simulink model "OneLeg_VR_TouchInput"  (Simulink 7.3)
settings: Solver=ode15s  StartTime=0.0  StopTime=inf  RelTol=1e-3
PreLoadFcn:
  | init_hopper
PostLoadFcn:
  | vrmfunc('FnOpen', [bdroot, '/Data Display and Analysis/VR Sink']);
undefined symbols (not defined in the file or in its folder): body, ctrl, ground, leg, sfuntraj, sigbuilder_block, Traj
libraries: mblibv1 x27, dspmtrx3 x8, simulink x4, vrlib x1
(part 1 of 2)
settings Model: Creator=grouleau  LastModifiedBy=grouleau
settings DataIOCC: SignalLoggingName=log
settings OptimizationCC: InitFltsAndDblsToZero=on
settings SimMechanicsCC: VisSampleTime=0.0667  AnimationDelay=0  LastVizWinPosition=[619 721 850 247]  CamPosition=[3.67411;0.656374;23.7815;]  CamTarget=[3.67411;0.656374;0;]  CamUpVector=[0;1;0;]  CamHeight=2.15758  VisBackgroundColor=[0.9;0.9;0.95;]  DefaultBodyColor=[1;0;0;]

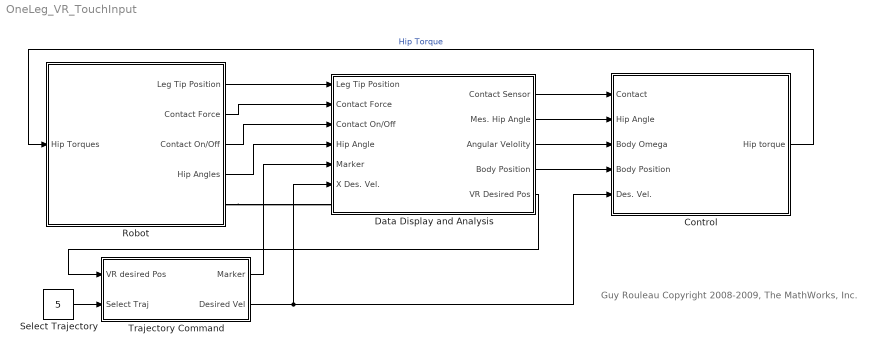
== system OneLeg_VR_TouchInput ==
  note: Guy Rouleau
      | Copyright 2008-2009, The MathWorks, Inc.
  Control : Subsystem
  Data Display and Analysis : Subsystem
  Robot : Subsystem
  Select Trajectory : Constant  Value=5  OutDataType=sfix(16)  OutScaling=2^0
  Trajectory Command : Subsystem
  wires:
  Robot/1(Leg Tip Position) -> Data Display and Analysis/1(Leg Tip Position)
  Control/1(Hip torque) -> Robot/1(Hip Torques)  "Hip Torque"
  Data Display and Analysis/3(Angular Velolity) -> Control/3(Body Omega)
  Robot/4(Hip Angles) -> Data Display and Analysis/4(Hip Angle)
  Trajectory Command/2(Desired Vel) -> Data Display and Analysis/6(X Des. Vel.), Control/5(Des. Vel.)
  Data Display and Analysis/4(Body Position) -> Control/4(Body Position)
  Data Display and Analysis/2(Mes. Hip Angle) -> Control/2(Hip Angle)
  Trajectory Command/1(Marker) -> Data Display and Analysis/5(Marker)
  Select Trajectory/1 -> Trajectory Command/2(Select Traj)
  Robot/3(Contact On/Off) -> Data Display and Analysis/3(Contact On/Off)
  Robot/2(Contact Force) -> Data Display and Analysis/2(Contact Force)
  Data Display and Analysis/5(VR Desired Pos) -> Trajectory Command/1(VR desired Pos)
  Data Display and Analysis/1(Contact Sensor) -> Control/1(Contact)
  connections:
  Robot/RConn1 -- Data Display and Analysis/LConn1

== system OneLeg_VR_TouchInput/Control ==
  Contact : Inport
  Hip Angle : Inport  Port=2
  Body Omega : Inport  Port=3
  Body Position : Inport  Port=4
  Des. Vel. : Inport  Port=5
  Body Angle Control : Subsystem
  Integrator : Integrator  LimitOutput=on  UpperSaturationLimit=1  LowerSaturationLimit=-1
  Logical Operator1 : Logic  Operator=NOT  AllPortsSameDT=off  OutDataTypeMode=boolean  OutDataTypeStr=boolean
  Motion analysis : Subsystem
  Saturation : Saturate  UpperLimit=ctrl.MaxHipTorque  LowerLimit=-ctrl.MaxHipTorque  OutDataType=sfix(16)  OutScaling=2^0
  Switch : Switch  Criteria=u2 ~= 0  OutDataType=sfix(16)  OutScaling=2^0
  Velocity Control : Subsystem
  Hip torque : Outport
  wires:
  Contact/1 -> Motion analysis/1(Contact), Switch/2, Logical Operator1/1, Body Angle Control/Enable
  Motion analysis/4(X stance) -> Velocity Control/4(X stance)
  Motion analysis/3(Body Vel) -> Velocity Control/3(Body Vel)
  Saturation/1 -> Hip torque/1
  Motion analysis/2(T up) -> Velocity Control/2(Air Duration)
  Hip Angle/1 -> Motion analysis/2(Hip Angle)
  Integrator/1 -> Motion analysis/3(Body Angle)
  Motion analysis/5(Leg Length) -> Velocity Control/5(Leg Length)
  Motion analysis/6(Hip Angle o) -> Velocity Control/6(Hip Angle)
  Motion analysis/1(Body Angle o) -> Body Angle Control/1(Theta), Velocity Control/1(Body Angle)
  Logical Operator1/1 -> Velocity Control/Enable
  Switch/1 -> Saturation/1
  Body Angle Control/1(Cmd) -> Switch/1
  Body Omega/1 -> Body Angle Control/2(Omega body), Integrator/1
  Velocity Control/1(Cmd) -> Switch/3
  Des. Vel./1 -> Motion analysis/4(Des. Vel.)
  Body Position/1 -> Motion analysis/5(Body Position)
  Motion analysis/7(Comp Des. Vel.) -> Velocity Control/7(Desired Velocity)
  Motion analysis/8(Comp Des. Pos.) -> Velocity Control/8(Desired Position)
  Motion analysis/9(Comp Body Pos.) -> Velocity Control/9(Body Pos)

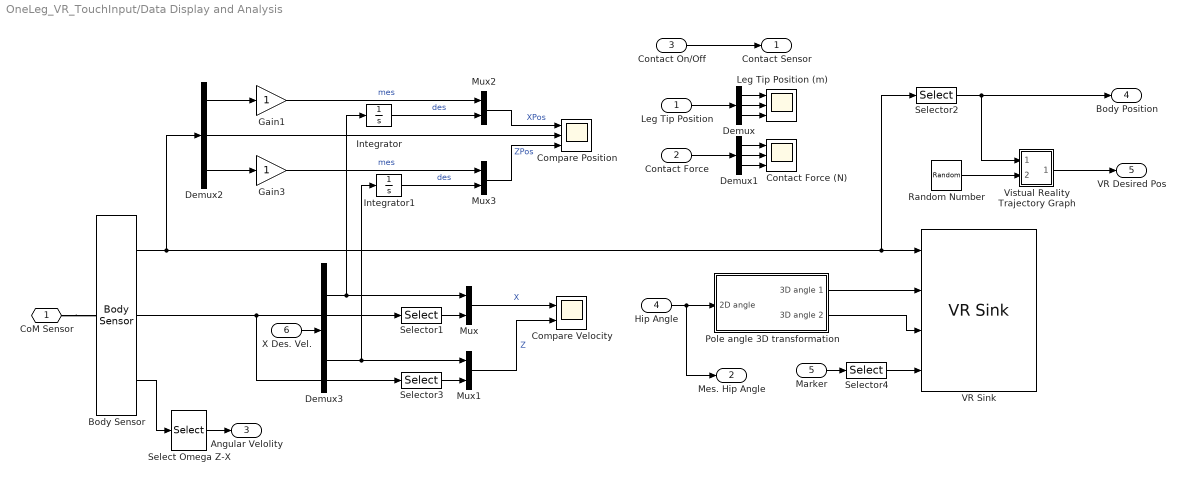
== system OneLeg_VR_TouchInput/Data Display and Analysis ==
  Leg Tip Position : Inport
  Contact Force : Inport  Port=2
  Contact On/Off : Inport  Port=3
  Hip Angle : Inport  Port=4
  Marker : Inport  Port=5
  X Des. Vel. : Inport  Port=6
  Body Sensor : mblibv1/Sensors &  Actuators/Body Sensor  DialogController=MECH.DynMechDlgSource  SystemSampleTime=-1  UpdateFromCAD=off  PhysicalDomain=Mechanical  PortType=blob  Muxed=off  Pose=off  Angle=on  AngleUnits=deg  ArcVelocity=on  ArcVelocityUnits=rad/s  ArcAcceleration=off  ArcAccelerationUnits=deg/s^2  CoordPosition=on  CoordPositionUnits=m  Velocity=on  VelocityUnits=m/s  Acceleration=off  AccelerationUnits=m/s^2  Quaternion=on  QuaternionDT=off  QuaternionDDT=off  QuaternionUnits=off  OutputVector=[1]  ActiveIO=on  Width=9  DialogClass=MechanicalSensorBlock  ReferenceFrame=Absolute (World)
  Compare Position : Scope  NumInputPorts=3
      settings: TimeRange=60  YMin=0~0.6~-1  YMax=4~1.15~1  SaveName=BodyData
  Compare Velocity : Scope  NumInputPorts=2
      settings: TimeRange=60  YMin=0.65~-1  YMax=1.2~1  SaveName=ScopeData10
  Contact Force (N) : Scope  NumInputPorts=3
      settings: TimeRange=2.5  YMin=-60000~0~-1  YMax=20000~20000~1
  Demux : Demux  Outputs=3
  Demux1 : Demux  Outputs=3
  Demux2 : Demux  Outputs=3
  Demux3 : Demux  Outputs=2
  Gain1 : Gain  ParameterDataType=sfix(16)  ParameterScaling=2^0  OutDataType=sfix(16)  OutScaling=2^0
  Gain3 : Gain  ParameterDataType=sfix(16)  ParameterScaling=2^0  OutDataType=sfix(16)  OutScaling=2^0
  Integrator : Integrator
  Integrator1 : Integrator
  Leg Tip Position (m) : Scope  NumInputPorts=3
      settings: YMin=-1~-0.05~-1  YMax=1~0.25~1  SaveName=FootData1
  Mux{,1..3} (4 alike) : Mux  Inputs=2
  Pole angle 3D transformation : Subsystem
  Random Number : RandomNumber  Mean=[0 0]  Variance=[5 5]  Seed=[0 5]  SampleTime=3
  Select Omega Z-X : Selector  InputPortWidth=3  IndexOptions=Index vector (dialog)  Indices=[3 1]  OutputSizes=1
  Selector1 : Selector  InputPortWidth=3  IndexOptions=Index vector (dialog)  Indices=[1 ]  OutputSizes=1
  Selector2 : Selector  InputPortWidth=3  IndexOptions=Index vector (dialog)  Indices=[1 3 ]  OutputSizes=1
  Selector3 : Selector  InputPortWidth=3  IndexOptions=Index vector (dialog)  Indices=[3 ]  OutputSizes=1
  Selector4 : Selector  InputPortWidth=3  IndexOptions=Index vector (dialog)  Indices=[1 3 2 ]  OutputSizes=1
  VR Sink : vrlib/VR Sink  InstantiateOnLoad=on  SampleTime=1/15  ViewEnable=on  RemoteChange=off  RemoteView=off  FieldsWritten=Pendulum.translation.3.1.double#Pole1.rotation.4.1.double#Pole2.rotation.4.1.double#Marker.translation.3.1.double  WorldFileName=robotVR.wrl  WorldDescription=Hopping Robot  AutoView=off  VideoDimensions=[]  FigureProperties="{'Position', 'Name', 'Viewpoint', 'CameraBound', 'CameraDirection', 'CameraPosition', 'CameraUpVector', 'ZoomFactor', 'Antialiasing', 'Headlight', 'Lighting', 'NavPanel', 'StatusBar', 'ToolBar', 'Textures', 'Transparency', 'Wireframe', 'NavZones', 'NavMode', 'NavSpeed', 'Record2DCompressMethod', 'Record2DCompressQuality', 'Record2D', 'Record2DFileName', 'Record2DFPS'; [5.0000000000000000e+000  9.2000000000000000e+001  5.7600000000000000e+002  3.8000000000000000e+002], 'Hopping Robot', 'Close view', 'on', [0.0000000000000000e+000  0.0000000000000000e+000 -1.0000000000000000e+000], [0.0000000000000000e+000  0.0000000000000000e+000  0.0000000000000000e+000], [0.0000000000000000e+000  1.0000000000000000e+000  0.0000000000000000e+000], [1.0000000000000000e+000], 'off', 'on', 'on', 'halfbar', 'on', 'on', 'on', 'on', 'off', 'off', 'examine', 'normal', 'auto', [7.5000000000000000e+001], 'off', '%f_anim_%n.avi', [1.5000000000000000e+001]}"
  Vistual Reality Trajectory Graph : Subsystem  LoadFcn=sfuntraj([],[],[],'LoadBlock')  StartFcn=sfuntraj([],[],[],'Start')  StopFcn=sfuntraj([],[],[],'Stop')  mask(Trajectory scope.){xmin=-10, xmax=10, ymin=-10, ymax=10, Ts=0.2, mode=VR sensor}
      mask prompts: xmin "x-min:"; xmax "x-max:"; ymin "y-min:"; ymax "y-max:"; Ts "Sample time:"; mode "Setpoint mode"
      mask help: Trajectory scope using MATLAB graph window. Enter plotting ranges.
      settings: CopyFcn=sfuntraj([],[],[],'CopyBlock')  DeleteFcn=sfuntraj([],[],[],'DeleteBlock')  NameChangeFcn=sfuntraj([],[],[],'NameChange')
      mask Help: This block can be used to explore limit cycles. Look at the m-file sfuntraj.m to see how it works.
      mask StyleString: edit,edit,edit,edit,edit,popup(Mouse|Input signal|VR sensor)
      mask Display: plot([.05 .95 .95 .05 .05],[.45 .45 .95 .95 .45], 0.5+cos(0:0.1:2*pi)*0.3,0.7+sin(0:0.1:2*pi)*0.2)
  CoM Sensor : PMIOPort  Port=1  Side=Left
  Contact Sensor : Outport
  Mes. Hip Angle : Outport  Port=2
  Angular Velolity : Outport  Port=3
  Body Position : Outport  Port=4
  VR Desired Pos : Outport  Port=5
  wires:
  Mux/1 -> Compare Velocity/1  "X"
  Selector1/1 -> Mux/2
  Body Sensor/2 -> Selector1/1, Selector3/1
  Mux1/1 -> Compare Velocity/2  "Z"
  Selector3/1 -> Mux1/2
  Body Sensor/1 -> Demux2/1, VR Sink/1, Selector2/1
  Demux3/1 -> Mux/1, Integrator/1
  Demux3/2 -> Mux1/1, Integrator1/1
  Body Sensor/3 -> Select Omega Z-X/1
  Hip Angle/1 -> Pole angle 3D transformation/1(2D angle), Mes. Hip Angle/1
  Pole angle 3D transformation/1(3D angle 1) -> VR Sink/2
  Pole angle 3D transformation/2(3D angle 2) -> VR Sink/3
  Marker/1 -> Selector4/1
  Integrator/1 -> Mux2/2  "des"
  Demux2/1 -> Gain1/1
  Integrator1/1 -> Mux3/2  "des"
  Demux2/3 -> Gain3/1
  Demux2/2 -> Compare Position/2
  Mux2/1 -> Compare Position/1  "XPos"
  Mux3/1 -> Compare Position/3  "ZPos"
  Gain1/1 -> Mux2/1  "mes"
  Gain3/1 -> Mux3/1  "mes"
  Selector2/1 -> Body Position/1, Vistual Reality Trajectory Graph/1(data)
  Select Omega Z-X/1 -> Angular Velolity/1
  Selector4/1 -> VR Sink/4
  Demux/1 -> Leg Tip Position (m)/1
  Demux/2 -> Leg Tip Position (m)/2
  Demux/3 -> Leg Tip Position (m)/3
  Leg Tip Position/1 -> Demux/1
  Contact Force/1 -> Demux1/1
  Demux1/1 -> Contact Force (N)/1
  Demux1/2 -> Contact Force (N)/2
  Demux1/3 -> Contact Force (N)/3
  X Des. Vel./1 -> Demux3/1
  Contact On/Off/1 -> Contact Sensor/1
  Random Number/1 -> Vistual Reality Trajectory Graph/2(setpoint)
  Vistual Reality Trajectory Graph/1(mouse) -> VR Desired Pos/1
  connections:
  CoM Sensor/RConn1 -- Body Sensor/LConn1

== system OneLeg_VR_TouchInput/Robot ==
  Hip Torques : Inport
  Body : Subsystem
  Hip : Subsystem
  Leg : mblibv1/Bodies/Body  DialogController=MECH.DynMechDlgSource  PhysicalDomain=mechanical  SubClassName=Unknown  LeftPortType=workingframe  RightPortType=workingframe  LConnTagsString=CS1  RConnTagsString=CS2  UpdateFromCAD=off  DialogClass=MechanicalBodyBlock  Mass=leg.mass  MassUnits=kg  InertiaUnits=kg*m^2  Inertia=leg.inertia  Shape=Cylinder  ShapeDims=[1 1]  ShapeUnits=m  ShapeUse=false  Density=1  DensityUnits=kg/m^3  DensityUse=false  GraphicsMode=1  BodyColorSelMode=MACHINE_DEFAULT  BodyColor=[0.5 0.5 0.5]  AttachedToCS=1  CG="Left$CG$[0 -leg.length/3  0]$CS1$CS1$m$[0 0 0]$Euler X-Y-Z$rad$Adjoining$false$none"  WorkingFrames=Left$CS1$[0 0 0]$Adjoining$Adjoining$m$[0 0 0]$Euler X-Y-Z$deg$CG$true$none#Right$CS2$[0 -leg.length 0]$CS1$CS1$m$[0 0 0]$Euler X-Y-Z$deg$CS1$true$none  CGPos="[0 -leg.length/3  0]"  CGRot=[0 0 0]  CS0Pos=[]  CS0Rot=[]  CS1Pos=[0 0 0]  CS1Rot=[0 0 0]  CS2Pos=[0 -leg.length 0]  CS2Rot=[0 0 0]  CS3Pos=[]  CS3Rot=[]  CS4Pos=[]  CS4Rot=[]  CS5Pos=[]  CS5Rot=[]  CS6Pos=[]  CS6Rot=[]  CS7Pos=[]  CS7Rot=[]  CS8Pos=[]  CS8Rot=[]  CS9Pos=[]  CS9Rot=[]  CS10Pos=[]  CS10Rot=[]  CS11Pos=[]  CS11Rot=[]  CS12Pos=[]  CS12Rot=[]  CS13Pos=[]  CS13Rot=[]  CS14Pos=[]  CS14Rot=[]  CS15Pos=[]  CS15Rot=[]  CS16Pos=[]  CS16Rot=[]  CS17Pos=[]  CS17Rot=[]  CS18Pos=[]  CS18Rot=[]  CS19Pos=[]  CS19Rot=[]  CS20Pos=[]  CS20Rot=[]
  Leg Tip and Contact Dynamics : Subsystem
  Simplified Hydraulic Actuator : Subsystem
  Spring : Subsystem
  ComSensor : PMIOPort  Port=1  Side=Right
  Leg Tip Position : Outport
  Contact Force : Outport  Port=2
  Contact On/Off : Outport  Port=3
  Hip Angles : Outport  Port=4
  wires:
  Spring/1(Length) -> Simplified Hydraulic Actuator/1(Spring Length)
  Hip Torques/1 -> Hip/1(Torques)
  Hip/1(Hip Angles) -> Hip Angles/1
  Leg Tip and Contact Dynamics/1(Pos) -> Leg Tip Position/1
  Leg Tip and Contact Dynamics/2(Contact Force2) -> Contact Force/1  "Force (N)"
  Leg Tip and Contact Dynamics/3(Contact) -> Contact On/Off/1  "Contact"
  connections:
  Body/RConn1 -- Hip/LConn1
  Hip/RConn1 -- Leg/LConn1
  Leg/RConn1 -- Simplified Hydraulic Actuator/LConn1
  Spring/RConn1 -- Leg Tip and Contact Dynamics/LConn1
  Simplified Hydraulic Actuator/RConn1 -- Spring/LConn1
  ComSensor/RConn1 -- Body/RConn2

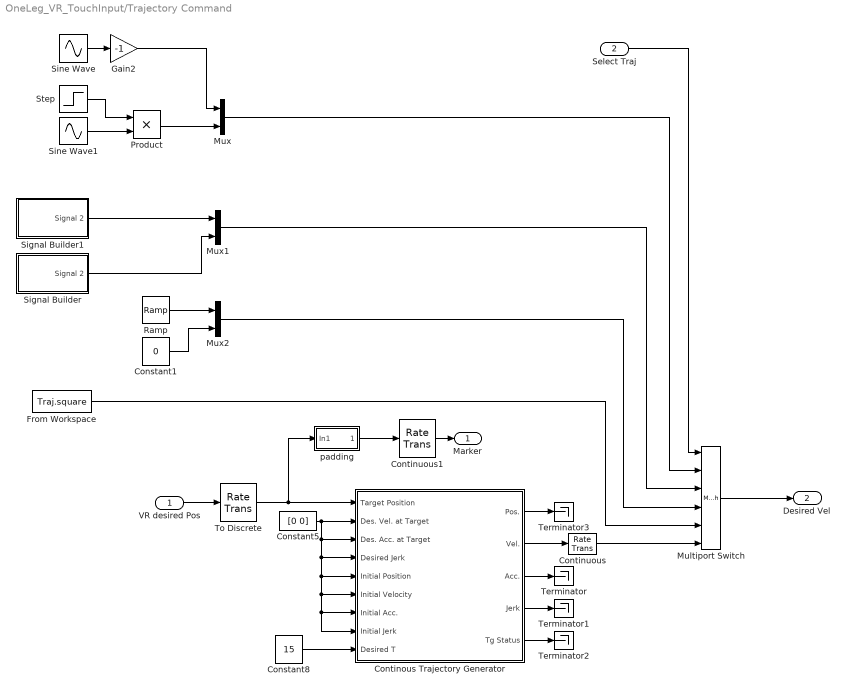
== system OneLeg_VR_TouchInput/Trajectory Command ==
  VR desired Pos : Inport  OutDataType=sfix(16)  OutScaling=2^0
  Select Traj : Inport  Port=2  OutDataType=sfix(16)  OutScaling=2^0
  Constant1 : Constant  Value=0  OutDataType=sfix(16)  OutScaling=2^0
  Constant5 : Constant  Value=[0 0]  OutDataType=sfix(16)  OutScaling=2^0  SampleTime=.01
  Constant8 : Constant  Value=15  OutDataType=sfix(16)  OutScaling=2^0  SampleTime=.01
  Continous Trajectory Generator : Subsystem  mask(Discrete Trajectory Generator: 5th Order Polynomial){UpdateLimit=0.0001, max_acc=50, maxv=.25, st=.01, Synchro=on}
      mask prompts: UpdateLimit "Treshold for Trajectory Update"; max_acc "Maximum acceleration"; maxv "Maximum velocity"; st "Sample time"; Synchro "Activate Synchronization"
      mask help:
      | Generates a 5th order polynomial trajectory between the current output and the desired position, velocity and acceleration. The motion will be executed in the requested trajectory time.
      | - The trajectory is updated when desired position changes
      | - This blocks accepts vectorized inputs.
      | - The input signals should have the same sampling time as the block.
      | - The motion will start one time step after the block is enabled and will be completed within the requested time if possible.
      mask Display: disp('7th Order\nPolynomial')
  Continuous : RateTransition  OutPortSampleTime=0
  Continuous1 : RateTransition  OutPortSampleTime=0
  From Workspace : FromWorkspace  VariableName=Traj.square  SampleTime=0  OutputAfterFinalValue=Holding final value
  Gain2 : Gain  Gain=-1  ParameterDataType=sfix(16)  ParameterScaling=2^0  OutDataType=sfix(16)  OutScaling=2^0
  Multiport Switch : MultiPortSwitch  Inputs=5  OutDataType=sfix(16)  OutScaling=2^0
  Mux : Mux  Inputs=2
  Mux1 : Mux  Inputs=2
  Mux2 : Mux  Inputs=2
  Product : Product  OutDataType=sfix(16)  OutScaling=2^0  RndMeth=Zero
  Ramp : simulink/Sources/Ramp  SystemSampleTime=-1  slope=.01  start=5  X0=0
  Signal Builder : Subsystem  Tag=STV Subsys  LoadFcn=sigbuilder_block('load');  StartFcn=sigbuilder_block('start');  StopFcn=sigbuilder_block('stop');  ClipboardFcn=sigbuilder_block('clipboard');  mask(Sigbuilder block){}
      mask help: Sigbuilder GUI
      mask init:
      | if ~strcmp(get_param(bdroot(gcbh),'SimulationStatus'),'stopped') tuvar = sigbuilder_block('maskInit'); end
      settings: CopyFcn=sigbuilder_block('copy');  DeleteFcn=sigbuilder_block('delete');  ModelCloseFcn=sigbuilder_block('modelClose');  PreSaveFcn=sigbuilder_block('preSave');  NameChangeFcn=sigbuilder_block('namechange');  OpenFcn=sigbuilder_block('open',[537.75 129 550.5 399.75 ]);  CloseFcn=sigbuilder_block('close');
      mask Display: plot(0,0,100,100,[10,10,40,40,10],[80,20,20,80,80],[40,10],[50,50], [40,27,10],[65,72,56],[40,25,25,10],[28,28,43,43]);
  Signal Builder1 : Subsystem  Tag=STV Subsys  LoadFcn=sigbuilder_block('load');  StartFcn=sigbuilder_block('start');  StopFcn=sigbuilder_block('stop');  ClipboardFcn=sigbuilder_block('clipboard');  mask(Sigbuilder block){}
      mask help: Sigbuilder GUI
      mask init:
      | if ~strcmp(get_param(bdroot(gcbh),'SimulationStatus'),'stopped') tuvar = sigbuilder_block('maskInit'); end
      settings: CopyFcn=sigbuilder_block('copy');  DeleteFcn=sigbuilder_block('delete');  ModelCloseFcn=sigbuilder_block('modelClose');  PreSaveFcn=sigbuilder_block('preSave');  NameChangeFcn=sigbuilder_block('namechange');  OpenFcn=sigbuilder_block('open',[537.75 129 550.5 399.75 ]);  CloseFcn=sigbuilder_block('close');
      mask Display: plot(0,0,100,100,[10,10,40,40,10],[80,20,20,80,80],[40,10],[50,50], [40,27,10],[65,72,56],[40,25,25,10],[28,28,43,43]);
  Sine Wave : Sin  Amplitude=Traj.circle.A  Bias=0  Frequency=Traj.circle.omega  Phase=0  Samples=10  SampleTime=0  Offset=0
  Sine Wave1 : Sin  Amplitude=Traj.circle.A  Bias=0  Frequency=Traj.circle.omega  Phase=pi/2  Samples=10  SampleTime=0  Offset=0
  Step : Step  Time=Traj.circle.starttime  SampleTime=0
  Terminator{,1..3} (4 alike) : Terminator
  To Discrete : RateTransition  OutPortSampleTime=.01
  padding : Subsystem
  Marker : Outport
  Desired Vel : Outport  Port=2
  wires:
  Sine Wave/1 -> Gain2/1
  Sine Wave1/1 -> Product/2
  Step/1 -> Product/1
  Gain2/1 -> Mux/1
  Signal Builder1/1(Signal 2) -> Mux1/1
  Signal Builder/1(Signal 2) -> Mux1/2
  Product/1 -> Mux/2
  Multiport Switch/1 -> Desired Vel/1
  Select Traj/1 -> Multiport Switch/1
  Mux/1 -> Multiport Switch/2
  Ramp/1 -> Mux2/1
  Constant1/1 -> Mux2/2
  Mux2/1 -> Multiport Switch/4
  Mux1/1 -> Multiport Switch/3
  From Workspace/1 -> Multiport Switch/5
  Constant5/1 -> Continous Trajectory Generator/2(Des. Vel. at Target), Continous Trajectory Generator/3(Des. Acc. at Target), Continous Trajectory Generator/4(Desired Jerk), Continous Trajectory Generator/5(Initial Position), Continous Trajectory Generator/6(Initial Velocity), Continous Trajectory Generator/7(Initial Acc.), Continous Trajectory Generator/8(Initial Jerk)
  Constant8/1 -> Continous Trajectory Generator/9(Desired T)
  Continous Trajectory Generator/2(Vel.) -> Continuous/1
  Continous Trajectory Generator/3(Acc.) -> Terminator/1
  Continous Trajectory Generator/4(Jerk) -> Terminator1/1
  Continous Trajectory Generator/5(Tg Status) -> Terminator2/1
  Continous Trajectory Generator/1(Pos.) -> Terminator3/1
  Continuous/1 -> Multiport Switch/6
  VR desired Pos/1 -> To Discrete/1
  padding/1(Out1) -> Continuous1/1
  Continuous1/1 -> Marker/1
  To Discrete/1 -> padding/1(In1), Continous Trajectory Generator/1(Target Position)

== system OneLeg_VR_TouchInput/Control/Body Angle Control ==
  Theta : Inport
  Omega body : Inport  Port=2
  Enable : EnablePort
  Omega Gain : Gain  Gain=ctrl.angle.Kv  ParameterDataType=sfix(16)  ParameterScaling=2^0  OutDataType=sfix(16)  OutScaling=2^0
  Position Gain : Gain  Gain=ctrl.angle.Kp  ParameterDataType=sfix(16)  ParameterScaling=2^0  OutDataType=sfix(16)  OutScaling=2^0
  Sum6 : Sum  Inputs=|++  OutDataType=sfix(16)  OutScaling=2^0
  Cmd : Outport
  wires:
  Sum6/1 -> Cmd/1
  Omega body/1 -> Omega Gain/1
  Theta/1 -> Position Gain/1
  Omega Gain/1 -> Sum6/2
  Position Gain/1 -> Sum6/1

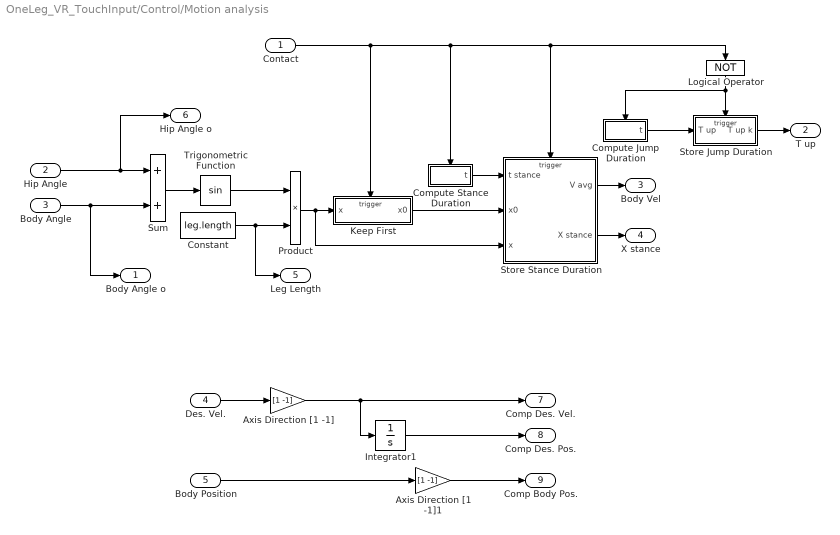
== system OneLeg_VR_TouchInput/Control/Motion analysis ==
  Contact : Inport
  Hip Angle : Inport  Port=2
  Body Angle : Inport  Port=3
  Des. Vel. : Inport  Port=4
  Body Position : Inport  Port=5
  Axis Direction [1 -1] : Gain  Gain=[1 -1]  ParameterDataType=sfix(16)  ParameterScaling=2^0  OutDataType=sfix(16)  OutScaling=2^0
  Axis Direction [1 -1]1 : Gain  Gain=[1 -1]  ParameterDataType=sfix(16)  ParameterScaling=2^0  OutDataType=sfix(16)  OutScaling=2^0
  Compute Jump Duration : Subsystem
  Compute Stance Duration : Subsystem
  Constant : Constant  Value=leg.length  OutDataType=sfix(16)  OutScaling=2^0
  Integrator1 : Integrator
  Keep First : Subsystem  TreatAsAtomicUnit=on
  Logical Operator : Logic  Operator=NOT  AllPortsSameDT=off  OutDataTypeMode=boolean  OutDataTypeStr=boolean
  Product : Product  OutDataType=sfix(16)  OutScaling=2^0  RndMeth=Zero
  Store Jump Duration : Subsystem  TreatAsAtomicUnit=on
  Store Stance Duration : Subsystem  TreatAsAtomicUnit=on
  Sum : Sum  OutDataType=sfix(16)  OutScaling=2^0
  Trigonometric Function : Trigonometry
  Body Angle o : Outport
  T up : Outport  Port=2
  Body Vel : Outport  Port=3
  X stance : Outport  Port=4
  Leg Length : Outport  Port=5
  Hip Angle o : Outport  Port=6
  Comp Des. Vel. : Outport  Port=7
  Comp Des. Pos. : Outport  Port=8
  Comp Body Pos. : Outport  Port=9
  wires:
  Hip Angle/1 -> Hip Angle o/1, Sum/1
  Body Angle/1 -> Body Angle o/1, Sum/2
  Sum/1 -> Trigonometric Function/1
  Trigonometric Function/1 -> Product/1
  Product/1 -> Keep First/1(x), Store Stance Duration/3(x)
  Keep First/1(x0) -> Store Stance Duration/2(x0)
  Compute Stance Duration/1(t) -> Store Stance Duration/1(t stance)
  Logical Operator/1 -> Compute Jump Duration/Enable, Store Jump Duration/Trigger
  Compute Jump Duration/1(t) -> Store Jump Duration/1(T up)
  Contact/1 -> Keep First/Trigger, Compute Stance Duration/Enable, Logical Operator/1, Store Stance Duration/Trigger
  Store Jump Duration/1(T up k) -> T up/1
  Store Stance Duration/1(V avg) -> Body Vel/1
  Store Stance Duration/2(X stance) -> X stance/1
  Constant/1 -> Product/2, Leg Length/1
  Des. Vel./1 -> Axis Direction [1 -1]/1
  Body Position/1 -> Axis Direction [1 -1]1/1
  Axis Direction [1 -1]/1 -> Integrator1/1, Comp Des. Vel./1
  Integrator1/1 -> Comp Des. Pos./1
  Axis Direction [1 -1]1/1 -> Comp Body Pos./1

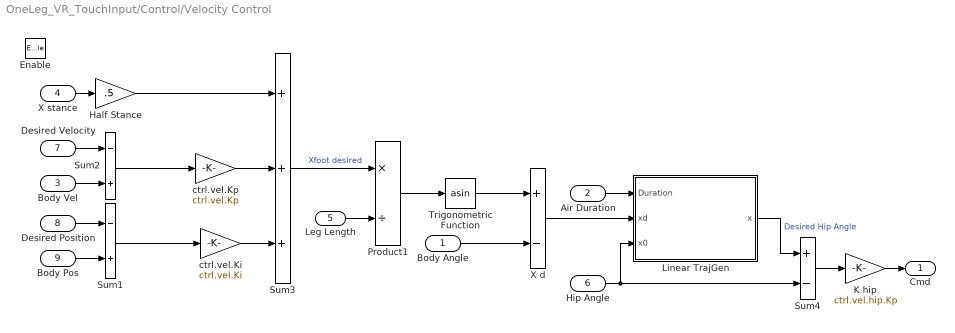
== system OneLeg_VR_TouchInput/Control/Velocity Control ==
  Body Angle : Inport
  Air Duration : Inport  Port=2
  Body Vel : Inport  Port=3
  X stance : Inport  Port=4
  Leg Length : Inport  Port=5
  Hip Angle : Inport  Port=6
  Desired Velocity : Inport  Port=7
  Desired Position : Inport  Port=8
  Body Pos : Inport  Port=9
  Enable : EnablePort  StatesWhenEnabling=reset
  Half Stance : Gain  Gain=.5  ParameterDataType=sfix(16)  ParameterScaling=2^0  OutDataType=sfix(16)  OutScaling=2^0
  K hip : Gain  Gain=ctrl.vel.hip.Kp  ParameterDataType=sfix(16)  ParameterScaling=2^0  OutDataType=sfix(16)  OutScaling=2^0
  Linear TrajGen : Subsystem
  Product1 : Product  Inputs=*/  OutDataType=sfix(16)  OutScaling=2^0  RndMeth=Zero
  Sum1 : Sum  Inputs=-+  OutDataType=sfix(16)  OutScaling=2^0
  Sum2 : Sum  Inputs=-+  OutDataType=sfix(16)  OutScaling=2^0
  Sum3 : Sum  Inputs=+++  OutDataType=sfix(16)  OutScaling=2^0
  Sum4 : Sum  Inputs=+-  OutDataType=sfix(16)  OutScaling=2^0
  Trigonometric Function : Trigonometry  Operator=asin
  X d : Sum  Inputs=+-  OutDataType=sfix(16)  OutScaling=2^0
  ctrl.vel.Ki : Gain  Gain=ctrl.vel.Ki  ParameterDataType=sfix(16)  ParameterScaling=2^0  OutDataType=sfix(16)  OutScaling=2^0
  ctrl.vel.Kp : Gain  Gain=ctrl.vel.Kp  ParameterDataType=sfix(16)  ParameterScaling=2^0  OutDataType=sfix(16)  OutScaling=2^0
  Cmd : Outport
  wires:
  Desired Velocity/1 -> Sum2/1
  X d/1 -> Linear TrajGen/2(xd)
  Leg Length/1 -> Product1/2
  Body Vel/1 -> Sum2/2
  Body Angle/1 -> X d/2
  Product1/1 -> Trigonometric Function/1
  Sum3/1 -> Product1/1  "Xfoot desired"
  ctrl.vel.Kp/1 -> Sum3/2
  Sum2/1 -> ctrl.vel.Kp/1
  Half Stance/1 -> Sum3/1
  Trigonometric Function/1 -> X d/1
  X stance/1 -> Half Stance/1
  Sum4/1 -> K hip/1
  K hip/1 -> Cmd/1
  Air Duration/1 -> Linear TrajGen/1(Duration)
  Linear TrajGen/1(x) -> Sum4/1  "Desired Hip Angle"
  Hip Angle/1 -> Sum4/2, Linear TrajGen/3(x0)
  ctrl.vel.Ki/1 -> Sum3/3
  Body Pos/1 -> Sum1/2
  Desired Position/1 -> Sum1/1
  Sum1/1 -> ctrl.vel.Ki/1

== system OneLeg_VR_TouchInput/Data Display and Analysis/Pole angle 3D transformation ==
  2D angle : Inport  OutDataType=sfix(16)  OutScaling=2^0
  Axis 1 : Constant  Value=[ 1 0 0 ]  OutDataType=sfix(16)  OutScaling=2^0
  Axis 2 : Constant  Value=[ 0 0 -1 ]  OutDataType=sfix(16)  OutScaling=2^0
  Demux3 : Demux  Outputs=2
  Mux6 : Mux  Inputs=2
  Mux7 : Mux  Inputs=2
  3D angle 1 : Outport  OutDataType=sfix(16)  OutScaling=2^0
  3D angle 2 : Outport  Port=2  OutDataType=sfix(16)  OutScaling=2^0
  wires:
  Mux6/1 -> 3D angle 2/1
  Demux3/2 -> Mux6/2
  Demux3/1 -> Mux7/2
  Mux7/1 -> 3D angle 1/1
  2D angle/1 -> Demux3/1
  Axis 2/1 -> Mux6/1
  Axis 1/1 -> Mux7/1

== system OneLeg_VR_TouchInput/Data Display and Analysis/Vistual Reality Trajectory Graph ==
  data : Inport  OutDataType=sfix(16)  OutScaling=2^0
  setpoint : Inport  Port=2  OutDataType=sfix(16)  OutScaling=2^0
  Mux : Mux  Inputs=2
  Setpoint : Constant  Value="[0.97482        1.42]"  OutDataType=sfix(16)  OutScaling=2^0
  sfuntraj : S-Function  FunctionName=sfuntraj  Parameters=[xmin xmax ymin ymax], Ts, mode  EnableBusSupport=off
  mouse : Outport  OutDataType=sfix(16)  OutScaling=2^0
  wires:
  Setpoint/1 -> mouse/1
  Mux/1 -> sfuntraj/1
  data/1 -> Mux/1
  setpoint/1 -> Mux/2

== system OneLeg_VR_TouchInput/Robot/Body ==
  Ground : mblibv1/Bodies/Ground  DialogController=MECH.DynMechDlgSource  SystemSampleTime=-1  UpdateFromCAD=off  LeftPortType=env  RightPortType=workingframe  PhysicalDomain=Mechanical  DialogClass=GroundBlock  CoordPosition=[0 0 0]  CoordPositionUnits=m  StateVectorMgrId=-1  MachineId=[0 0]  ShowEnvPort=on
  Ground for viz : mblibv1/Bodies/Body  DialogController=MECH.DynMechDlgSource  PhysicalDomain=mechanical  SubClassName=Unknown  LeftPortType=workingframe  RightPortType=workingframe  LConnTagsString=CS1  RConnTagsString=CS2  UpdateFromCAD=off  DialogClass=MechanicalBodyBlock  Mass=1  MassUnits=kg  InertiaUnits=kg*m^2  Inertia=eye(3)  Shape=Cylinder  ShapeDims=[1 1]  ShapeUnits=m  ShapeUse=false  Density=1  DensityUnits=kg/m^3  DensityUse=false  GraphicsMode=MACHINE_DEFAULT  BodyColorSelMode=COLORPALETTE  BodyColor=[0 0 0]  AttachedToCS=CG  CG=Left$CG$[0 0 0]$WORLD$WORLD$m$[0 0 0]$Euler X-Y-Z$deg$WORLD$false$none  WorkingFrames=Left$CS1$[0 0 0]$CG$CG$m$[0 0 0]$Euler X-Y-Z$deg$WORLD$true$none#Right$CS2$[0 0 0]$CG$CG$m$[0 0 0]$Euler X-Y-Z$deg$WORLD$true$none#Right$CS3$[0 0 0]$CG$CG$m$[0 0 0]$Euler X-Y-Z$deg$WORLD$false$none#Right$CS4$[0 -0.2 0]$CG$CG$m$[0 0 0]$Euler X-Y-Z$deg$WORLD$false$none#Right$CS6$[20 0 0]$CG$CG$m$[0 0 0]$Euler X-Y-Z$deg$WORLD$false$none#Right$CS5$[20 -0.2 0]$CG$CG$m$[0 0 0]$Euler X-Y-Z$deg$WORLD$false$none  CGPos=[0 0 0]  CGRot=[0 0 0]  CS0Pos=[]  CS0Rot=[]  CS1Pos=[0 0 0]  CS1Rot=[0 0 0]  CS2Pos=[0 0 0]  CS2Rot=[0 0 0]  CS3Pos=[0 0 0]  CS3Rot=[0 0 0]  CS4Pos=[0 -0.2 0]  CS4Rot=[0 0 0]  CS5Pos=[20 -0.2 0]  CS5Rot=[0 0 0]  CS6Pos=[20 0 0]  CS6Rot=[0 0 0]  CS7Pos=[]  CS7Rot=[]  CS8Pos=[]  CS8Rot=[]  CS9Pos=[]  CS9Rot=[]  CS10Pos=[]  CS10Rot=[]  CS11Pos=[]  CS11Rot=[]  CS12Pos=[]  CS12Rot=[]  CS13Pos=[]  CS13Rot=[]  CS14Pos=[]  CS14Rot=[]  CS15Pos=[]  CS15Rot=[]  CS16Pos=[]  CS16Rot=[]  CS17Pos=[]  CS17Rot=[]  CS18Pos=[]  CS18Rot=[]  CS19Pos=[]  CS19Rot=[]  CS20Pos=[]  CS20Rot=[]
  Joint Initial Condition : mblibv1/Sensors &  Actuators/Joint Initial Condition  DialogController=MECH.DynMechDlgSource  SystemSampleTime=-1  UpdateFromCAD=off  PhysicalDomain=mechanical  DialogClass=InitialConditionBlock  InitialConditions=P1$false$0$m$deg$0$m/s$deg/s#P2$true$0.98$m$deg$0$m/s$deg/s#P3$false$0$m$deg$0$m/s$deg/s#R1$false$0$m$deg$0$m/s$deg/s#R2$false$0$m$deg$0$m/s$deg/s#R3$false$0$m$deg$0$m/s$deg/s#S$false$0$m$deg$0$m/s$deg/s  P1PIC=0  P1VIC=0  P2PIC=0.98  P2VIC=0  P3PIC=0  P3VIC=0  R1PIC=0  R1VIC=0  R2PIC=0  R2VIC=0  R3PIC=0  R3VIC=0  SPIC=0  SVIC=0
  Machine Environment : mblibv1/Bodies/Machine Environment  Tag=Factory ground  DialogController=MECH.DialogSource  SystemSampleTime=-1  PortType=env  PhysicalDomain=Mechanical  DialogTemplateClass=MECH.MachineEnvironment  SyncWhenCopied=off  Gravity=[0 -9.81 0]  GravityUnits=m/s^2  GravityAsSignal=off  Dimensionality=3D Only  AnalysisType=Forward dynamics  LinearAssemblyTolerance=1e-3  LinearAssemblyToleranceUnits=m  AngularAssemblyTolerance=1e-3  AngularAssemblyToleranceUnits=rad  ConstraintSolverType=Stabilizing  ConstraintRelTolerance=1e-4  ConstraintAbsTolerance=1e-4  UseRobustSingularityHandling=off  RedundancyAnalysisToleranceType=Automatically select tolerance  RedundancyAnalysisTolerance=1e-14  StatePerturbationType=Adaptive  PerturbationSize=1e-3  VisualizeMachine=on  BodyVisualizationType=Use model default body geometries  BodyColorSelMode=Use model default  DefaultBodyColor=[1 0 0]
  Robot Body : mblibv1/Bodies/Body  DialogController=MECH.DynMechDlgSource  PhysicalDomain=mechanical  SubClassName=Unknown  LeftPortType=workingframe  RightPortType=workingframe  LConnTagsString=CS1  RConnTagsString=CG|CS6  UpdateFromCAD=off  DialogClass=MechanicalBodyBlock  Mass=body.mass  MassUnits=kg  InertiaUnits=kg*m^2  Inertia=body.inertia  Shape=Cylinder  ShapeDims=[1 1]  ShapeUnits=m  ShapeUse=false  Density=1  DensityUnits=kg/m^3  DensityUse=false  GraphicsMode=1  BodyColorSelMode=MACHINE_DEFAULT  BodyColor=[0.5 0.5 0.5]  AttachedToCS=1  CG="Right$CG$[0 0  0]$CS1$CS1$m$[0 0 0]$Euler X-Y-Z$rad$Adjoining$true$none"  WorkingFrames="Left$CS1$[ 0 0 0]$Adjoining$Adjoining$m$[0 0 0]$Euler X-Y-Z$deg$CG$true$none#Right$CS6$[ 0 0 0]$CS1$CS1$m$[0 0 0]$Euler X-Y-Z$deg$CG$true$none#Right$CS2$[  body.xdim body.ydim body.zdim]$CS1$CS1$m$[0 0 0]$Euler X-Y-Z$deg$CG$false$none#Right$CS4$[  -body.xdim body.ydim body.zdim]$CS1$CS1$m$[0 0 0]$Euler X-Y-Z$deg$CG$false$none#Right$CS5$[  -body.xdim -body.ydim body.zdim]$CS1$CS1$m$[0 0 0]$Euler X-Y-Z$deg$CG$false$none#Right$CS7$[  body.xdim -body.ydim body.zdim]$CS1$CS1$m$[0 0 0]$Euler X-Y-Z$deg$CG$false$none#Right$CS3$[  body.xdim body.ydim -body.zdim]$CS1$CS1$m$[0 0 0]$Euler X-Y-Z$rad$Adjoining$false$none#Right$CS10$[  -body.xdim body.ydim -body.zdim]$CS1$CS1$m$[0 0 0]$Euler X-Y-Z$rad$Adjoining$false$none#Right$CS9$[  -body.xdim -body.ydim -body.zdim]$CS1$CS1$m$[0 0 0]$Euler X-Y-Z$rad$Adjoining$false$none#Right$CS8$[  body.xdim -body.ydim -body.zdim]$CS1$CS1$m$[0 0 0]$Euler X-Y-Z$rad$Adjoining$false$none"  CGPos="[0 0  0]"  CGRot=[0 0 0]  CS0Pos=[]  CS0Rot=[]  CS1Pos=[ 0 0 0]  CS1Rot=[0 0 0]  CS2Pos="[  body.xdim body.ydim body.zdim]"  CS2Rot=[0 0 0]  CS3Pos="[  body.xdim body.ydim -body.zdim]"  CS3Rot=[0 0 0]  CS4Pos="[  -body.xdim body.ydim body.zdim]"  CS4Rot=[0 0 0]  CS5Pos="[  -body.xdim -body.ydim body.zdim]"  CS5Rot=[0 0 0]  CS6Pos=[ 0 0 0]  CS6Rot=[0 0 0]  CS7Pos="[  body.xdim -body.ydim body.zdim]"  CS7Rot=[0 0 0]  CS8Pos="[  body.xdim -body.ydim -body.zdim]"  CS8Rot=[0 0 0]  CS9Pos="[  -body.xdim -body.ydim -body.zdim]"  CS9Rot=[0 0 0]  CS10Pos="[  -body.xdim body.ydim -body.zdim]"  CS10Rot=[0 0 0]  CS11Pos=[]  CS11Rot=[]  CS12Pos=[]  CS12Rot=[]  CS13Pos=[]  CS13Rot=[]  CS14Pos=[]  CS14Rot=[]  CS15Pos=[]  CS15Rot=[]  CS16Pos=[]  CS16Rot=[]  CS17Pos=[]  CS17Rot=[]  CS18Pos=[]  CS18Rot=[]  CS19Pos=[]  CS19Rot=[]  CS20Pos=[]  CS20Rot=[]
  Transition : mblibv1/Bodies/Body  DialogController=MECH.DynMechDlgSource  PhysicalDomain=mechanical  SubClassName=Unknown  LeftPortType=workingframe  RightPortType=workingframe  LConnTagsString=CS1  RConnTagsString=CS2  UpdateFromCAD=off  DialogClass=MechanicalBodyBlock  Mass=.001  MassUnits=kg  InertiaUnits=kg*m^2  Inertia=.00001*eye(3)  Shape=Cylinder  ShapeDims=[1 1]  ShapeUnits=m  ShapeUse=false  Density=1  DensityUnits=kg/m^3  DensityUse=false  GraphicsMode=1  BodyColorSelMode=MACHINE_DEFAULT  BodyColor=[0.5 0.5 0.5]  AttachedToCS=1  CG=Left$CG$[0 0 0]$WORLD$WORLD$m$[0 0 0]$Euler X-Y-Z$deg$WORLD$false$none  WorkingFrames=Left$CS1$[0 0 0]$CG$CG$m$[0 0 0]$Euler X-Y-Z$deg$WORLD$true$none#Right$CS2$[0 0 0]$CG$CG$m$[0 0 0]$Euler X-Y-Z$deg$WORLD$true$none  CGPos=[0 0 0]  CGRot=[0 0 0]  CS0Pos=[]  CS0Rot=[]  CS1Pos=[0 0 0]  CS1Rot=[0 0 0]  CS2Pos=[0 0 0]  CS2Rot=[0 0 0]  CS3Pos=[]  CS3Rot=[]  CS4Pos=[]  CS4Rot=[]  CS5Pos=[]  CS5Rot=[]  CS6Pos=[]  CS6Rot=[]  CS7Pos=[]  CS7Rot=[]  CS8Pos=[]  CS8Rot=[]  CS9Pos=[]  CS9Rot=[]  CS10Pos=[]  CS10Rot=[]  CS11Pos=[]  CS11Rot=[]  CS12Pos=[]  CS12Rot=[]  CS13Pos=[]  CS13Rot=[]  CS14Pos=[]  CS14Rot=[]  CS15Pos=[]  CS15Rot=[]  CS16Pos=[]  CS16Rot=[]  CS17Pos=[]  CS17Rot=[]  CS18Pos=[]  CS18Rot=[]  CS19Pos=[]  CS19Rot=[]  CS20Pos=[]  CS20Rot=[]
  Translation : mblibv1/Joints/Custom Joint  DialogController=MECH.DynMechDlgSource  PhysicalDomain=mechanical  SubClassName=custom_joint  LeftPortType=blob  RightPortType=blob  LConnTagsString=__newl0|SA1  RConnTagsString=__newr0  UpdateFromCAD=off  NumSAPorts=1  CutJoint=off  MarkAsCut=off  Primitives=prismatic  PrimitiveProps=P1$World$[1 0 0]$Prismatic#P2$World$[0 1 0]$Prismatic#P3$World$[0 0 1]$Prismatic  DialogClass=JointBlock  R1Axis=[]  R2Axis=[]  R3Axis=[]  P1Axis=[1 0 0]  P2Axis=[0 1 0]  P3Axis=[0 0 1]  SAxis=[]
  Universal : mblibv1/Joints/Universal  DialogController=MECH.DynMechDlgSource  PhysicalDomain=mechanical  SubClassName=Unknown  LeftPortType=blob  RightPortType=blob  LConnTagsString=__newl0  RConnTagsString=__newr0  UpdateFromCAD=off  NumSAPorts=0  CutJoint=off  MarkAsCut=off  Primitives=prismatic  PrimitiveProps=R1$World$[1 0 0]$revolute#R2$World$[0 0 1]$revolute  DialogClass=JointBlock  R1Axis=[1 0 0]  R2Axis=[0 0 1]
  Weld : mblibv1/Joints/Weld  DialogController=MECH.DynMechDlgSource  PhysicalDomain=mechanical  SubClassName=Unknown  LeftPortType=blob  RightPortType=blob  LConnTagsString=__newl0  RConnTagsString=__newr0  UpdateFromCAD=off  NumSAPorts=0  CutJoint=off  MarkAsCut=off  Primitives=weld  PrimitiveProps=W$WORLD$[0 0 0]$weld  DialogClass=JointBlock  WAxis=[0 0 0]
  Hip : PMIOPort  Port=1  Side=Right
  CoM Sensor : PMIOPort  Port=2  Side=Right
  connections:
  Machine Environment/RConn1 -- Ground/LConn1
  Joint Initial Condition/RConn1 -- Translation/LConn2
  Hip/RConn1 -- Robot Body/RConn1
  CoM Sensor/RConn1 -- Robot Body/RConn2
  Translation/RConn1 -- Transition/LConn1
  Transition/RConn1 -- Universal/LConn1
  Universal/RConn1 -- Robot Body/LConn1
  Ground for viz/RConn1 -- Translation/LConn1
  Ground/RConn1 -- Weld/LConn1
  Weld/RConn1 -- Ground for viz/LConn1

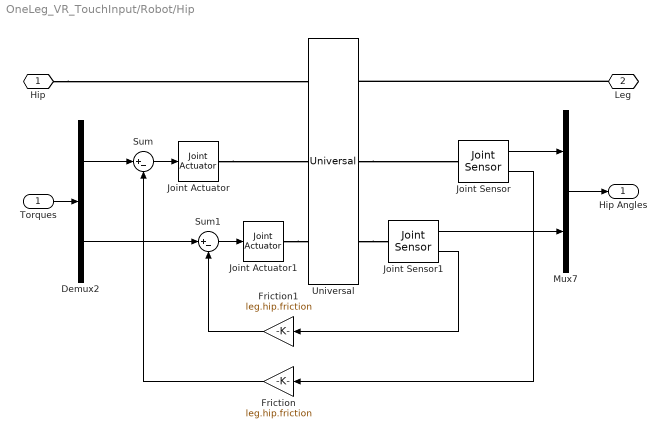
== system OneLeg_VR_TouchInput/Robot/Hip ==
  Torques : Inport
  Demux2 : Demux  Outputs=2
  Friction : Gain  Gain=leg.hip.friction  ParameterDataType=sfix(16)  ParameterScaling=2^0  OutDataType=sfix(16)  OutScaling=2^0
  Friction1 : Gain  Gain=leg.hip.friction  ParameterDataType=sfix(16)  ParameterScaling=2^0  OutDataType=sfix(16)  OutScaling=2^0
  Joint Actuator : mblibv1/Sensors &  Actuators/Joint Actuator  DialogController=MECH.DynMechDlgSource  SystemSampleTime=-1  UpdateFromCAD=off  PhysicalDomain=Mechanical  PortType=blob  ActuationStyle=Force  AngleUnits=deg  ArcVelocityUnits=deg/s  ArcAccelerationUnits=deg/s^2  CoordPositionUnits=m  VelocityUnits=m/s  AccelerationUnits=m/s^2  ForceUnits=N  TorqueUnits=N*m  ActiveIO=on  Width=1  DialogClass=MechanicalActuatorBlock  Primitive=R1  ReferenceFrame=Absolute (World)
  Joint Actuator1 : mblibv1/Sensors &  Actuators/Joint Actuator  DialogController=MECH.DynMechDlgSource  SystemSampleTime=-1  UpdateFromCAD=off  PhysicalDomain=Mechanical  PortType=blob  ActuationStyle=Force  AngleUnits=deg  ArcVelocityUnits=deg/s  ArcAccelerationUnits=deg/s^2  CoordPositionUnits=m  VelocityUnits=m/s  AccelerationUnits=m/s^2  ForceUnits=N  TorqueUnits=N*m  ActiveIO=on  Width=1  DialogClass=MechanicalActuatorBlock  Primitive=R2  ReferenceFrame=Absolute (World)
  Joint Sensor : mblibv1/Sensors &  Actuators/Joint Sensor  DialogController=MECH.DynMechDlgSource  SystemSampleTime=-1  UpdateFromCAD=off  PhysicalDomain=Mechanical  PortType=blob  Muxed=off  Pose=off  Angle=on  AngleUnits=rad  ArcVelocity=on  ArcVelocityUnits=rad/s  ArcAcceleration=off  ArcAccelerationUnits=deg/s^2  CoordPosition=on  CoordPositionUnits=m  Velocity=off  VelocityUnits=m/s  Acceleration=off  AccelerationUnits=m/s^2  Quaternion=on  QuaternionDT=off  QuaternionDDT=off  QuaternionUnits=off  OutputVector=[1]  ActiveIO=on  Width=2  DialogClass=MechanicalSensorBlock  Primitive=R1  Force=off  ForceUnits=N  Torque=off  TorqueUnits=N*m  ReferenceFrame=Absolute (World)  ReactionSensedSide=Base  ReactionReferenceFrame=Local (Body CS)  ReactionForce=off  ReactionForceUnits=N  ReactionMoment=off  ReactionMomentUnits=N*m
  Joint Sensor1 : mblibv1/Sensors &  Actuators/Joint Sensor  DialogController=MECH.DynMechDlgSource  SystemSampleTime=-1  UpdateFromCAD=off  PhysicalDomain=Mechanical  PortType=blob  Muxed=off  Pose=off  Angle=on  AngleUnits=rad  ArcVelocity=on  ArcVelocityUnits=rad/s  ArcAcceleration=off  ArcAccelerationUnits=deg/s^2  CoordPosition=on  CoordPositionUnits=m  Velocity=off  VelocityUnits=m/s  Acceleration=off  AccelerationUnits=m/s^2  Quaternion=on  QuaternionDT=off  QuaternionDDT=off  QuaternionUnits=off  OutputVector=[1]  ActiveIO=on  Width=2  DialogClass=MechanicalSensorBlock  Primitive=R2  Force=off  ForceUnits=N  Torque=off  TorqueUnits=N*m  ReferenceFrame=Absolute (World)  ReactionSensedSide=Base  ReactionReferenceFrame=Local (Body CS)  ReactionForce=off  ReactionForceUnits=N  ReactionMoment=off  ReactionMomentUnits=N*m
  Mux7 : Mux  Inputs=2
  Sum : Sum  Inputs=|+-  OutDataType=sfix(16)  OutScaling=2^0
  Sum1 : Sum  Inputs=|+-  OutDataType=sfix(16)  OutScaling=2^0
  Universal : mblibv1/Joints/Universal  DialogController=MECH.DynMechDlgSource  PhysicalDomain=mechanical  SubClassName=Unknown  LeftPortType=blob  RightPortType=blob  LConnTagsString=__newl0|SA1|SA2  RConnTagsString=__newr0|SA1|SA2  UpdateFromCAD=off  NumSAPorts=4  CutJoint=off  MarkAsCut=off  Primitives=prismatic  PrimitiveProps="R1$Base$[0 0 1]$revolute#R2$Base$[1 0  0]$revolute"  DialogClass=JointBlock  R1Axis=[0 0 1]  R2Axis="[1 0  0]"
  Hip : PMIOPort  Port=1  Side=Left
  Leg : PMIOPort  Port=2  Side=Right
  Hip Angles : Outport
  wires:
  Joint Sensor/2 -> Friction/1
  Sum/1 -> Joint Actuator/1
  Friction/1 -> Sum/2
  Demux2/1 -> Sum/1
  Joint Sensor/1 -> Mux7/1
  Joint Sensor1/1 -> Mux7/2
  Sum1/1 -> Joint Actuator1/1
  Demux2/2 -> Sum1/1
  Friction1/1 -> Sum1/2
  Joint Sensor1/2 -> Friction1/1
  Torques/1 -> Demux2/1
  Mux7/1 -> Hip Angles/1
  connections:
  Joint Actuator/RConn1 -- Universal/LConn2
  Universal/RConn2 -- Joint Sensor/LConn1
  Hip/RConn1 -- Universal/LConn1
  Leg/RConn1 -- Universal/RConn1
  Universal/RConn3 -- Joint Sensor1/LConn1
  Joint Actuator1/RConn1 -- Universal/LConn3

== system OneLeg_VR_TouchInput/Robot/Leg Tip and Contact Dynamics ==
  Compare To Constant1 : simulink/Logic and Bit Operations/Compare To Constant  SystemSampleTime=-1  relop=<=  const=0  LogicOutDataTypeMode=uint8  ZeroCross=off
  Contact Force : Subsystem
  Leg Tip : mblibv1/Bodies/Body  DialogController=MECH.DynMechDlgSource  PhysicalDomain=mechanical  SubClassName=Unknown  LeftPortType=workingframe  RightPortType=workingframe  LConnTagsString=CG  RConnTagsString=CS2  UpdateFromCAD=off  DialogClass=MechanicalBodyBlock  Mass=0.01  MassUnits=kg  InertiaUnits=kg*m^2  Inertia=0.0001*eye(3)  Shape=Cylinder  ShapeDims=[1 1]  ShapeUnits=m  ShapeUse=false  Density=1  DensityUnits=kg/m^3  DensityUse=false  GraphicsMode=1  BodyColorSelMode=MACHINE_DEFAULT  BodyColor=[0.5 0.5 0.5]  AttachedToCS=1  CG=Left$CG$[0 0 0 ]$CS2$CS2$m$[0 0 0]$Euler X-Y-Z$deg$WORLD$true$none  WorkingFrames=Right$CS2$[0 0 0]$Adjoining$Adjoining$m$[0 0 0]$Euler X-Y-Z$deg$WORLD$true$none  CGPos=[0 0 0 ]  CGRot=[0 0 0]  CS0Pos=[]  CS0Rot=[]  CS1Pos=[]  CS1Rot=[]  CS2Pos=[0 0 0]  CS2Rot=[0 0 0]  CS3Pos=[]  CS3Rot=[]  CS4Pos=[]  CS4Rot=[]  CS5Pos=[]  CS5Rot=[]  CS6Pos=[]  CS6Rot=[]  CS7Pos=[]  CS7Rot=[]  CS8Pos=[]  CS8Rot=[]  CS9Pos=[]  CS9Rot=[]  CS10Pos=[]  CS10Rot=[]  CS11Pos=[]  CS11Rot=[]  CS12Pos=[]  CS12Rot=[]  CS13Pos=[]  CS13Rot=[]  CS14Pos=[]  CS14Rot=[]  CS15Pos=[]  CS15Rot=[]  CS16Pos=[]  CS16Rot=[]  CS17Pos=[]  CS17Rot=[]  CS18Pos=[]  CS18Rot=[]  CS19Pos=[]  CS19Rot=[]  CS20Pos=[]  CS20Rot=[]
  Selector : Selector  InputPortWidth=3  IndexOptions=Index vector (dialog)  Indices=[2]  OutputSizes=1
  Tip : PMIOPort  Port=1  Side=Left
  Pos : Outport
  Contact Force2 : Outport  Port=2  OutDataType=sfix(16)  OutScaling=2^0
  Contact : Outport  Port=3
  wires:
  Selector/1 -> Compare To Constant1/1
  Compare To Constant1/1 -> Contact/1
  Contact Force/1(Position) -> Selector/1, Pos/1
  Contact Force/2(Contact Force) -> Contact Force2/1
  connections:
  Contact Force/RConn1 -- Leg Tip/LConn1
  Tip/RConn1 -- Leg Tip/RConn1

== system OneLeg_VR_TouchInput/Robot/Simplified Hydraulic Actuator ==
  Spring Length : Inport
  Body : mblibv1/Bodies/Body  DialogController=MECH.DynMechDlgSource  PhysicalDomain=mechanical  SubClassName=Unknown  LeftPortType=workingframe  RightPortType=workingframe  LConnTagsString=CS1  RConnTagsString=CS2  UpdateFromCAD=off  DialogClass=MechanicalBodyBlock  Mass=0.001  MassUnits=kg  InertiaUnits=kg*m^2  Inertia=.0001*eye(3)  Shape=Cylinder  ShapeDims=[1 1]  ShapeUnits=m  ShapeUse=false  Density=1  DensityUnits=kg/m^3  DensityUse=false  GraphicsMode=1  BodyColorSelMode=MACHINE_DEFAULT  BodyColor=[0.5 0.5 0.5]  AttachedToCS=1  CG=Left$CG$[0 0 0]$CS1$CS1$m$[0 0 0]$Euler X-Y-Z$deg$WORLD$false$none  WorkingFrames=Left$CS1$[0 0 0]$Adjoining$Adjoining$m$[0 0 0]$Euler X-Y-Z$deg$WORLD$true$none#Right$CS2$[0 0 0]$CG$CG$m$[0 0 0]$Euler X-Y-Z$deg$WORLD$true$none  CGPos=[0 0 0]  CGRot=[0 0 0]  CS0Pos=[]  CS0Rot=[]  CS1Pos=[0 0 0]  CS1Rot=[0 0 0]  CS2Pos=[0 0 0]  CS2Rot=[0 0 0]  CS3Pos=[]  CS3Rot=[]  CS4Pos=[]  CS4Rot=[]  CS5Pos=[]  CS5Rot=[]  CS6Pos=[]  CS6Rot=[]  CS7Pos=[]  CS7Rot=[]  CS8Pos=[]  CS8Rot=[]  CS9Pos=[]  CS9Rot=[]  CS10Pos=[]  CS10Rot=[]  CS11Pos=[]  CS11Rot=[]  CS12Pos=[]  CS12Rot=[]  CS13Pos=[]  CS13Rot=[]  CS14Pos=[]  CS14Rot=[]  CS15Pos=[]  CS15Rot=[]  CS16Pos=[]  CS16Rot=[]  CS17Pos=[]  CS17Rot=[]  CS18Pos=[]  CS18Rot=[]  CS19Pos=[]  CS19Rot=[]  CS20Pos=[]  CS20Rot=[]
  Compare To Constant : simulink/Logic and Bit Operations/Compare To Constant  SystemSampleTime=-1  relop=>=  const=leg.actuator.Threshold  LogicOutDataTypeMode=uint8  ZeroCross=off
  Constant : Constant  Value=0  OutDataType=sfix(16)  OutScaling=2^0
  Constant1 : Constant  Value=leg.actuator.MaxLength  OutDataType=sfix(16)  OutScaling=2^0
  Friction : Gain  Gain=leg.actuator.c  ParameterDataType=sfix(16)  ParameterScaling=2^0  OutDataType=sfix(16)  OutScaling=2^0  SaturateOnIntegerOverflow=on  OutDataTypeStr=Inherit: Same as input  ParamDataTypeStr=Inherit: Same as input
  Joint Actuator1 : mblibv1/Sensors &  Actuators/Joint Actuator  DialogController=MECH.DynMechDlgSource  SystemSampleTime=-1  UpdateFromCAD=off  PhysicalDomain=Mechanical  PortType=blob  ActuationStyle=Force  AngleUnits=deg  ArcVelocityUnits=deg/s  ArcAccelerationUnits=deg/s^2  CoordPositionUnits=m  VelocityUnits=m/s  AccelerationUnits=m/s^2  ForceUnits=N  TorqueUnits=N-m  ActiveIO=on  Width=1  DialogClass=MechanicalActuatorBlock  Primitive=P1  ReferenceFrame=Absolute (World)
  Joint Sensor1 : mblibv1/Sensors &  Actuators/Joint Sensor  DialogController=MECH.DynMechDlgSource  SystemSampleTime=-1  UpdateFromCAD=off  PhysicalDomain=Mechanical  PortType=blob  Muxed=off  Pose=off  Angle=on  AngleUnits=deg  ArcVelocity=off  ArcVelocityUnits=deg/s  ArcAcceleration=off  ArcAccelerationUnits=deg/s^2  CoordPosition=on  CoordPositionUnits=m  Velocity=on  VelocityUnits=m/s  Acceleration=off  AccelerationUnits=m/s^2  Quaternion=on  QuaternionDT=off  QuaternionDDT=off  QuaternionUnits=off  OutputVector=[1]  ActiveIO=on  Width=2  DialogClass=MechanicalSensorBlock  Primitive=P1  Force=off  ForceUnits=N  Torque=off  TorqueUnits=N*m  ReferenceFrame=Absolute (World)  ReactionSensedSide=Base  ReactionReferenceFrame=Local (Body CS)  ReactionForce=off  ReactionForceUnits=N  ReactionMoment=off  ReactionMomentUnits=N*m
  Kp : Gain  Gain=leg.actuator.kp  ParameterDataType=sfix(16)  ParameterScaling=2^0  OutDataType=sfix(16)  OutScaling=2^0  SaturateOnIntegerOverflow=on  OutDataTypeStr=Inherit: Same as input  ParamDataTypeStr=Inherit: Same as input
  Leg Actuator : mblibv1/Joints/Prismatic  DialogController=MECH.DynMechDlgSource  PhysicalDomain=mechanical  SubClassName=Unknown  LeftPortType=blob  RightPortType=blob  LConnTagsString=__newl0|SA1  RConnTagsString=__newr0|SA1  UpdateFromCAD=off  NumSAPorts=2  CutJoint=off  MarkAsCut=off  Primitives=prismatic  PrimitiveProps=P1$Base$[0 1 0 ]$prismatic  DialogClass=JointBlock  P1Axis=[0 1 0 ]
  Sum1 : Sum  Inputs=--  OutDataType=sfix(16)  OutScaling=2^0  SaturateOnIntegerOverflow=on
  Sum2 : Sum  OutDataType=sfix(16)  OutScaling=2^0  SaturateOnIntegerOverflow=on
  Switch : Switch  Criteria=u2 ~= 0  OutDataType=sfix(16)  OutScaling=2^0
  Leg : PMIOPort  Port=1  Side=Left
  Spring : PMIOPort  Port=2  Side=Right
  wires:
  Spring Length/1 -> Compare To Constant/1
  Switch/1 -> Sum2/1
  Compare To Constant/1 -> Switch/2
  Constant1/1 -> Switch/1
  Constant/1 -> Switch/3
  Sum2/1 -> Kp/1
  Kp/1 -> Sum1/1
  Joint Sensor1/1 -> Sum2/2
  Friction/1 -> Sum1/2
  Sum1/1 -> Joint Actuator1/1
  Joint Sensor1/2 -> Friction/1
  connections:
  Body/RConn1 -- Spring/RConn1
  Body/LConn1 -- Leg Actuator/RConn1
  Leg/RConn1 -- Leg Actuator/LConn1
  Leg Actuator/RConn2 -- Joint Sensor1/LConn1
  Joint Actuator1/RConn1 -- Leg Actuator/LConn2

== system OneLeg_VR_TouchInput/Robot/Spring ==
  Firction : Gain  Gain=leg.damping  ParameterDataType=sfix(16)  ParameterScaling=2^0  OutDataType=sfix(16)  OutScaling=2^0  SaturateOnIntegerOverflow=on  OutDataTypeStr=Inherit: Same as input  ParamDataTypeStr=Inherit: Same as input
  Joint Actuator : mblibv1/Sensors &  Actuators/Joint Actuator  DialogController=MECH.DynMechDlgSource  SystemSampleTime=-1  UpdateFromCAD=off  PhysicalDomain=Mechanical  PortType=blob  ActuationStyle=Force  AngleUnits=deg  ArcVelocityUnits=deg/s  ArcAccelerationUnits=deg/s^2  CoordPositionUnits=m  VelocityUnits=m/s  AccelerationUnits=m/s^2  ForceUnits=N  TorqueUnits=N-m  ActiveIO=on  Width=1  DialogClass=MechanicalActuatorBlock  Primitive=P1  ReferenceFrame=Absolute (World)
  Joint Sensor : mblibv1/Sensors &  Actuators/Joint Sensor  DialogController=MECH.DynMechDlgSource  SystemSampleTime=-1  UpdateFromCAD=off  PhysicalDomain=Mechanical  PortType=blob  Muxed=off  Pose=off  Angle=on  AngleUnits=deg  ArcVelocity=off  ArcVelocityUnits=deg/s  ArcAcceleration=off  ArcAccelerationUnits=deg/s^2  CoordPosition=on  CoordPositionUnits=m  Velocity=on  VelocityUnits=m/s  Acceleration=off  AccelerationUnits=m/s^2  Quaternion=on  QuaternionDT=off  QuaternionDDT=off  QuaternionUnits=off  OutputVector=[1]  ActiveIO=on  Width=2  DialogClass=MechanicalSensorBlock  Primitive=P1  Force=off  ForceUnits=N  Torque=off  TorqueUnits=N*m  ReferenceFrame=Absolute (World)  ReactionSensedSide=Base  ReactionReferenceFrame=Local (Body CS)  ReactionForce=off  ReactionForceUnits=N  ReactionMoment=off  ReactionMomentUnits=N*m
  LegStiffness : Constant  Value=leg.stiffness  OutDataType=sfix(16)  OutScaling=2^0
  Prismatic : mblibv1/Joints/Prismatic  DialogController=MECH.DynMechDlgSource  PhysicalDomain=mechanical  SubClassName=Unknown  LeftPortType=blob  RightPortType=blob  LConnTagsString=__newl0|SA1  RConnTagsString=__newr0|SA1  UpdateFromCAD=off  NumSAPorts=2  CutJoint=off  MarkAsCut=off  Primitives=prismatic  PrimitiveProps=P1$Base$[0 1 0 ]$prismatic  DialogClass=JointBlock  P1Axis=[0 1 0 ]
  Product : Product  OutDataType=sfix(16)  OutScaling=2^0  RndMeth=Zero
  Sum : Sum  Inputs=--  OutDataType=sfix(16)  OutScaling=2^0  SaturateOnIntegerOverflow=on
  Spring : PMIOPort  Port=1  Side=Left
  Tip : PMIOPort  Port=2  Side=Right
  Length : Outport
  wires:
  Joint Sensor/1 -> Length/1, Product/2
  Joint Sensor/2 -> Firction/1
  Sum/1 -> Joint Actuator/1
  Firction/1 -> Sum/2
  Product/1 -> Sum/1
  LegStiffness/1 -> Product/1
  connections:
  Spring/RConn1 -- Prismatic/LConn1
  Tip/RConn1 -- Prismatic/RConn1
  Joint Sensor/LConn1 -- Prismatic/RConn2
  Joint Actuator/RConn1 -- Prismatic/LConn2
